simulink model "Regenerative_Braking_R2020b"  (R2019b)
settings: Solver=ode45  StartTime=0.0  StopTime=4  RelTol=1e-3  EnableMultiTasking=on
model workspace (MAT data in the model file):
  T = 20
libraries: powerlib x19
settings Model: Creator=Vikas  LastModifiedBy=merul
settings SolverCC: ZeroCrossAlgorithm=Adaptive
settings DataIOCC: LimitDataPoints=on  SaveFormat=Array  SignalLoggingSaveFormat=ModelDataLogs  ReturnWorkspaceOutputs=off
settings OptimizationCC: ExpressionDepthLimit=2147483647  LifeSpan=inf
settings DebuggingCC: UnderspecifiedInitializationDetection=Classic  MergeDetectMultiDrivingBlocksExec=none  IgnoredZcDiagnostic=none  SolverPrmCheckMsg=warning  FcnCallInpInsideContextMsg=warning  StateNameClashWarn=warning  SFUnexpectedBacktrackingDiag=warning  SFNoUnconditionalDefaultTransitionDiag=warning  SFExecutionAtInitializationDiag=none  ArithmeticOperatorsInVariantConditions=warning
settings HardwareCC: ProdBitPerPointer=32  ProdBitPerSizeT=32  ProdBitPerPtrDiffT=32  ProdLargestAtomicFloat=None  ProdIntDivRoundTo=Undefined  ProdEndianess=Unspecified  ProdWordSize=32  ProdHWDeviceType=32-bit Generic
settings ModelReferenceCC: PropagateSignalLabelsOutOfModel=off
settings SFSimCC: SimUseLocalCustomCode=off  CustomCodeUndefinedFunction=UseInterfaceOnly
settings RTWCC: RTWUseLocalCustomCode=off
settings CodeAppCC: StateflowObjectComments=on
settings GRTTargetCC: TargetLangStandard=C89/C90 (ANSI)  CombineOutputUpdateFcns=off  GRTInterface=on
settings ConfigComp: CovMetricSettings=dw  CovSaveCumulativeToWorkspaceVar=on  CovSaveSingleToWorkspaceVar=on  CovExternalEMLEnable=off

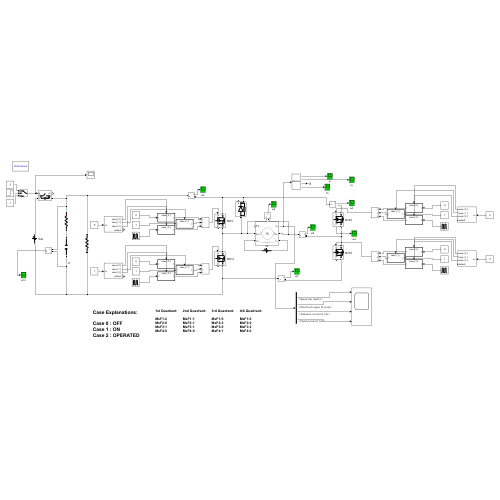
[thumbnail: Simulink's stored preview of the top-level diagram]
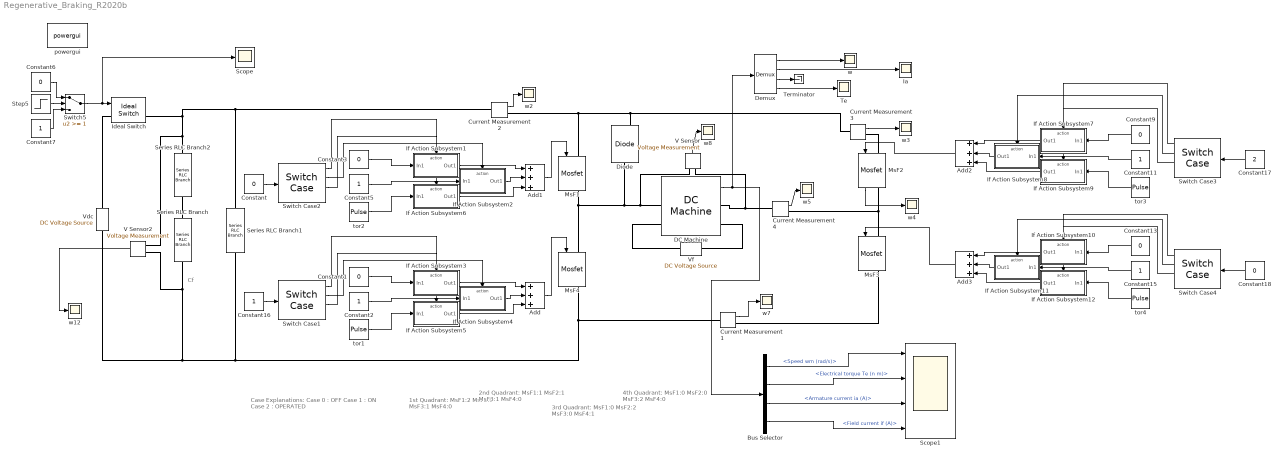
== system Regenerative_Braking_R2020b ==
  note: 1st Quadrant:
      |
      | MsF1:2
      | MsF2:0
      | MsF3:1
      | MsF4:0
  note: Case Explanations:
      |
      | Case 0 : OFF
      | Case 1 : ON
      | Case 2 : OPERATED
  note: Cf
  note: 2nd Quadrant:
      |
      | MsF1:1
      | MsF2:1
      | MsF3:1
      | MsF4:0
  note: 3rd Quadrant:
      |
      | MsF1:0
      | MsF2:2
      | MsF3:0
      | MsF4:1
  note: 4th Quadrant:
      |
      | MsF1:0
      | MsF2:0
      | MsF3:2
      | MsF4:0
  Add{,1..3} (4 alike) : Sum  Inputs=+++
  Bus Selector : BusSelector  OutputSignals=Speed wm (rad/s),Electrical torque Te (n m),Armature current ia (A),Field current if (A)
  Constant{,1,3,6,9,13,18} (7 alike) : Constant  Value=0
  Constant{2,5,7,11,15..16} (6 alike) : Constant
  Constant17 : Constant  Value=2
  Current Measurement{1..4} (4 alike) : powerlib/Measurements/Current Measurement  PhasorSimulation=off  OutputType=Complex  PSBequivalent=0
  DC Machine : powerlib/Machines/DC Machine  PresetModel=No  MechanicalLoad=Torque TL  FieldType=Wound  ShowDetailedParameters=on  MeasurementBus=off  RLa=[2.581 0.028]  RLf=[281.2 156]  Laf=0.9483  MachineConstant=Torque constant (N.m/A)  Ke=1.8  Kt=1.8  J=0.02215  Bm=0.002953  Tf=0.5161  w0=1  Ifinit=0.782361308677098  TsPowergui=0  TsBlock=-1
      settings: AttributesFormatString=\n
  Demux : Demux
      settings: DisplayOption=none
  Diode : powerlib/Power Electronics/Diode  Ron=0.001  Lon=0  Vf=0.8  IC=0  UseSnubber=0  Rs=500  Cs=250e-9  Measurements=on
  Ia : Scope
  Ideal Switch : powerlib/Power Electronics/Ideal Switch  Ron=0.001  Lon=0  IC=0  Rs=1e5  Cs=inf  Measurements=on
  If Action Subsystem1 : Subsystem  TreatAsAtomicUnit=on
  If Action Subsystem10 : Subsystem  TreatAsAtomicUnit=on
  If Action Subsystem11 : Subsystem  TreatAsAtomicUnit=on
  If Action Subsystem12 : Subsystem  TreatAsAtomicUnit=on
  If Action Subsystem2 : Subsystem  TreatAsAtomicUnit=on
  If Action Subsystem3 : Subsystem  TreatAsAtomicUnit=on
  If Action Subsystem4 : Subsystem  TreatAsAtomicUnit=on
  If Action Subsystem5 : Subsystem  TreatAsAtomicUnit=on
  If Action Subsystem6 : Subsystem  TreatAsAtomicUnit=on
  If Action Subsystem7 : Subsystem  TreatAsAtomicUnit=on
  If Action Subsystem8 : Subsystem  TreatAsAtomicUnit=on
  If Action Subsystem9 : Subsystem  TreatAsAtomicUnit=on
  MsF{1..4} (4 alike) : powerlib/Power Electronics/Mosfet  Ron=0.1  Lon=0  Rd=0.01  Vfd=0  IC=0  Rs=1e5  Cs=inf  Measurements=on
  Scope : Scope
  Scope1 : Scope  NumInputPorts=4
  Series RLC Branch : powerlib/Elements/Series RLC Branch  LConnTagsString=__new0  RConnTagsString=__new0  BranchType=C  Resistance=1  Inductance=1e-3  SetiL0=off  InitialCurrent=0  Capacitance=100e-6  Setx0=off  InitialVoltage=0  Measurements=None
  Series RLC Branch1 : powerlib/Elements/Series RLC Branch  LConnTagsString=__new0  RConnTagsString=__new0  BranchType=R  Resistance=10  Inductance=1e-3  SetiL0=off  InitialCurrent=0  Capacitance=1e-3  Setx0=off  InitialVoltage=0  Measurements=None
  Series RLC Branch2 : powerlib/Elements/Series RLC Branch  LConnTagsString=__new0  RConnTagsString=__new0  BranchType=R  Resistance=0.01  Inductance=1e-3  SetiL0=off  InitialCurrent=0  Capacitance=1e-3  Setx0=off  InitialVoltage=0  Measurements=None
  Step5 : Step  Time=1%3  SampleTime=0
  Switch Case{1..4} (4 alike) : SwitchCase  CaseConditions={0,1,2}
  Switch5 : Switch  Threshold=1
  Te : Scope
  Terminator : Terminator
  V Sensor : powerlib/Measurements/Voltage Measurement  PhasorSimulation=off  OutputType=Complex  PSBequivalent=0
  V Sensor2 : powerlib/Measurements/Voltage Measurement  PhasorSimulation=off  OutputType=Complex  PSBequivalent=0
  Vdc : powerlib/Electrical Sources/DC Voltage Source  Amplitude=220  Measurements=None
  Vf : powerlib/Electrical Sources/DC Voltage Source  Amplitude=220  Measurements=None
  powergui : powerlib/powergui  Priority=1  SimulationMode=Continuous  SampleTime=50e-6  frequency=60  Iterations=50  frequencyindice=0  Pbase=100e6  ErrMax=1e-4  UnitsV=kV  UnitsW=MW  buscounter=0  FunctionMessages=off  echomessages=off  EnableUseOfTLC=off  CurrentSourceSwitches=off  DisableSnubberDevices=off  DisableRonSwitches=off  DisableVfSwitches=off  DisplayEquations=off  AutomaticDiscreteSolvers=off  SolverType=Tustin/Backward Euler (TBE)  Interpol=off  ExternalGateDelay=off  methode=off  Ts=100  x0status=blocks  SPID=off  SwTol=0  HookPort=off  NonlinearTolerance=1e-4  nMaxIteration=100  ContinueOnMaxIteration=off  RestoreLinks=warning  ResistiveCurrentMeasurement=off  Frange=[0:2:500]  Ylog=off  Xlog=on  ShowGrid=off  save=off  variable=ZData  structure=0  ZoomFFT=off  StartTime=0.0  cycles=1  DisplayStyle=1  fundamental=60  FreqAxis=off  MaxFrequency=1000  frequencyindicesteady=1  RmsSteady=1  display=off
  tor{1..4} (4 alike) : DiscretePulseGenerator  PulseType=Time based  Period=0.0001  PulseWidth=80
  w{,2..5,7..8,12} (8 alike) : Scope
  wires:
  Demux/4 -> Te/1
  Demux/1 -> w/1
  Demux/2 -> Ia/1
  Demux/3 -> Terminator/1
  V Sensor/1 -> w8/1
  Current Measurement3/1 -> w3/1
  Current Measurement4/1 -> w5/1
  Current Measurement1/1 -> w7/1
  MsF2/1 -> w4/1
  V Sensor2/1 -> w12/1
  Constant6/1 -> Switch5/1
  Step5/1 -> Switch5/2
  Constant7/1 -> Switch5/3
  Switch5/1 -> Scope/1, Ideal Switch/1
  Current Measurement2/1 -> w2/1
  Bus Selector/2 -> Scope1/2  "<Electrical torque Te (n m)>"
  Bus Selector/3 -> Scope1/3  "<Armature current ia (A)>"
  Bus Selector/1 -> Scope1/1  "<Speed wm (rad/s)>"
  Bus Selector/4 -> Scope1/4  "<Field current if (A)>"
  DC Machine/1 -> Bus Selector/1, Demux/1
  Switch Case1/2 -> If Action Subsystem4/Action
  Switch Case1/1 -> If Action Subsystem3/Action
  Constant2/1 -> If Action Subsystem4/1(In1)
  Switch Case1/3 -> If Action Subsystem5/Action
  Constant1/1 -> If Action Subsystem3/1(In1)
  tor1/1 -> If Action Subsystem5/1(In1)
  If Action Subsystem5/1(Out1) -> Add/3
  If Action Subsystem4/1(Out1) -> Add/2
  If Action Subsystem3/1(Out1) -> Add/1
  Add/1 -> MsF4/1
  If Action Subsystem6/1(Out1) -> Add1/3
  If Action Subsystem1/1(Out1) -> Add1/1
  If Action Subsystem2/1(Out1) -> Add1/2
  Constant5/1 -> If Action Subsystem2/1(In1)
  Switch Case2/2 -> If Action Subsystem2/Action
  tor2/1 -> If Action Subsystem6/1(In1)
  Switch Case2/3 -> If Action Subsystem6/Action
  Switch Case2/1 -> If Action Subsystem1/Action
  Constant3/1 -> If Action Subsystem1/1(In1)
  If Action Subsystem9/1(Out1) -> Add2/3
  If Action Subsystem7/1(Out1) -> Add2/1
  If Action Subsystem8/1(Out1) -> Add2/2
  Constant11/1 -> If Action Subsystem8/1(In1)
  Switch Case3/2 -> If Action Subsystem8/Action
  tor3/1 -> If Action Subsystem9/1(In1)
  Switch Case3/3 -> If Action Subsystem9/Action
  Switch Case3/1 -> If Action Subsystem7/Action
  Constant9/1 -> If Action Subsystem7/1(In1)
  If Action Subsystem12/1(Out1) -> Add3/3
  If Action Subsystem10/1(Out1) -> Add3/1
  If Action Subsystem11/1(Out1) -> Add3/2
  Constant15/1 -> If Action Subsystem11/1(In1)
  Switch Case4/2 -> If Action Subsystem11/Action
  tor4/1 -> If Action Subsystem12/1(In1)
  Switch Case4/3 -> If Action Subsystem12/Action
  Switch Case4/1 -> If Action Subsystem10/Action
  Constant13/1 -> If Action Subsystem10/1(In1)
  Add1/1 -> MsF1/1
  Add2/1 -> MsF2/1
  Add3/1 -> MsF3/1
  Constant/1 -> Switch Case2/1
  Constant16/1 -> Switch Case1/1
  Constant18/1 -> Switch Case4/1
  Constant17/1 -> Switch Case3/1
  connections:
  DC Machine/LConn1 -- Diode/LConn1 -- MsF1/RConn1 -- MsF4/LConn1 -- V Sensor/LConn1
  Series RLC Branch/RConn1 -- Vdc/LConn1 -- Series RLC Branch1/RConn1 -- MsF4/RConn1 -- Current Measurement1/LConn1 -- V Sensor2/LConn2
  MsF1/LConn1 -- Diode/RConn1 -- Current Measurement3/LConn1 -- Current Measurement2/RConn1
  Ideal Switch/RConn1 -- Series RLC Branch1/LConn1 -- Current Measurement2/LConn1 -- V Sensor2/LConn1 -- Series RLC Branch2/LConn1
  MsF3/LConn1 -- MsF2/RConn1 -- Current Measurement4/RConn1
  DC Machine/LConn2 -- Vf/RConn1
  Current Measurement1/RConn1 -- MsF3/RConn1
  Series RLC Branch/LConn1 -- Series RLC Branch2/RConn1
  Current Measurement3/RConn1 -- MsF2/LConn1
  DC Machine/RConn1 -- Current Measurement4/LConn1 -- V Sensor/LConn2
  DC Machine/RConn2 -- Vf/LConn1
  Ideal Switch/LConn1 -- Vdc/RConn1

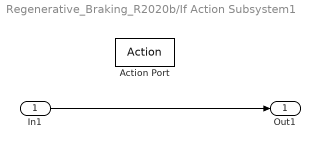
== system Regenerative_Braking_R2020b/If Action Subsystem1 ==
  In1 : Inport
  Action Port : ActionPort  ActionPortLabel=case [ 0 ]:
  Out1 : Outport
  wires:
  In1/1 -> Out1/1

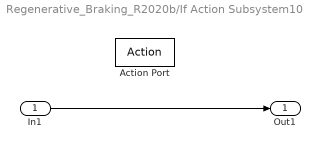
== system Regenerative_Braking_R2020b/If Action Subsystem10 ==
  In1 : Inport
  Action Port : ActionPort  ActionPortLabel=case [ 0 ]:
  Out1 : Outport
  wires:
  In1/1 -> Out1/1

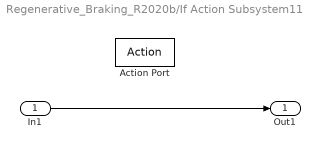
== system Regenerative_Braking_R2020b/If Action Subsystem11 ==
  In1 : Inport
  Action Port : ActionPort  ActionPortLabel=case [ 1 ]:
  Out1 : Outport
  wires:
  In1/1 -> Out1/1

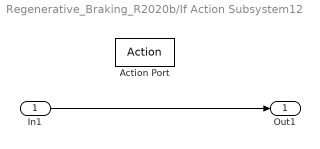
== system Regenerative_Braking_R2020b/If Action Subsystem12 ==
  In1 : Inport
  Action Port : ActionPort  ActionPortLabel=case [ 2 ]:
  Out1 : Outport
  wires:
  In1/1 -> Out1/1

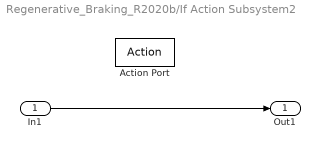
== system Regenerative_Braking_R2020b/If Action Subsystem2 ==
  In1 : Inport
  Action Port : ActionPort  ActionPortLabel=case [ 1 ]:
  Out1 : Outport
  wires:
  In1/1 -> Out1/1

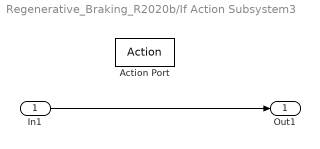
== system Regenerative_Braking_R2020b/If Action Subsystem3 ==
  In1 : Inport
  Action Port : ActionPort  ActionPortLabel=case [ 0 ]:
  Out1 : Outport
  wires:
  In1/1 -> Out1/1

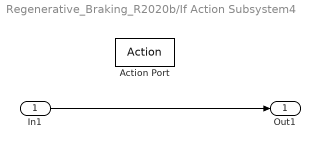
== system Regenerative_Braking_R2020b/If Action Subsystem4 ==
  In1 : Inport
  Action Port : ActionPort  ActionPortLabel=case [ 1 ]:
  Out1 : Outport
  wires:
  In1/1 -> Out1/1

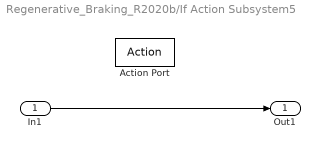
== system Regenerative_Braking_R2020b/If Action Subsystem5 ==
  In1 : Inport
  Action Port : ActionPort  ActionPortLabel=case [ 2 ]:
  Out1 : Outport
  wires:
  In1/1 -> Out1/1

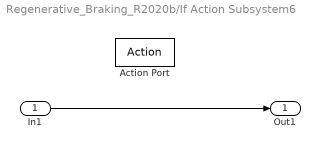
== system Regenerative_Braking_R2020b/If Action Subsystem6 ==
  In1 : Inport
  Action Port : ActionPort  ActionPortLabel=case [ 2 ]:
  Out1 : Outport
  wires:
  In1/1 -> Out1/1

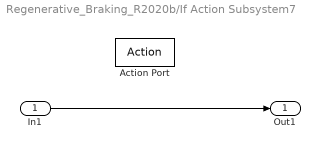
== system Regenerative_Braking_R2020b/If Action Subsystem7 ==
  In1 : Inport
  Action Port : ActionPort  ActionPortLabel=case [ 0 ]:
  Out1 : Outport
  wires:
  In1/1 -> Out1/1

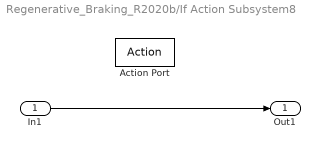
== system Regenerative_Braking_R2020b/If Action Subsystem8 ==
  In1 : Inport
  Action Port : ActionPort  ActionPortLabel=case [ 1 ]:
  Out1 : Outport
  wires:
  In1/1 -> Out1/1

== system Regenerative_Braking_R2020b/If Action Subsystem9 ==
  In1 : Inport
  Action Port : ActionPort  ActionPortLabel=case [ 2 ]:
  Out1 : Outport
  wires:
  In1/1 -> Out1/1
